simulink model "mod_liq2"  (R2016b)
settings: Solver=ode45  StartTime=0.0  StopTime=10.0  RelTol=1e-3  EnableMultiTasking=on
values from neighbouring files (symbols this model uses):
  Ar = 6*25.4    (= 152.4)    [param2NL.m]
  hmax = 16    [param2NL.m]
  k12 = 38    [param2NL.m]
  k2 = 11.5    [param2NL.m]
  qmax = 90    [param2NL.m]
  qmin = 0    [param2NL.m]
settings Model: Creator=Adolfo  LastModifiedBy=adolfobs
settings DataIOCC: LimitDataPoints=on  SaveFormat=Array  SignalLoggingSaveFormat=ModelDataLogs
settings OptimizationCC: ExpressionDepthLimit=2147483647  LifeSpan=inf
settings DebuggingCC: UnderspecifiedInitializationDetection=Classic  MergeDetectMultiDrivingBlocksExec=none  SolverPrmCheckMsg=warning  FcnCallInpInsideContextMsg=warning  StateNameClashWarn=warning  SFUnexpectedBacktrackingDiag=warning  SFNoUnconditionalDefaultTransitionDiag=warning  SFExecutionAtInitializationDiag=none
settings HardwareCC: ProdBitPerPointer=32  ProdBitPerSizeT=32  ProdBitPerPtrDiffT=32  ProdLargestAtomicFloat=None  ProdIntDivRoundTo=Undefined  ProdEndianess=Unspecified  ProdWordSize=32  ProdHWDeviceType=32-bit Generic
settings ModelReferenceCC: PropagateSignalLabelsOutOfModel=off
settings GRTTargetCC: TargetLangStandard=C89/C90 (ANSI)  GeneratePreprocessorConditionals=Disable all  CombineOutputUpdateFcns=off  GRTInterface=on
settings ConfigComp: CovMetricSettings=dw  CovHtmlReporting=on  CovSaveCumulativeToWorkspaceVar=on  CovSaveSingleToWorkspaceVar=on  CovExternalEMLEnable=off

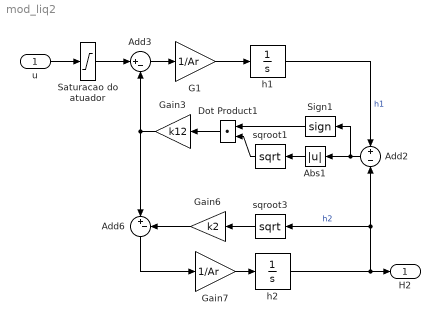
== system mod_liq2 ==
  u : Inport
  Abs1 : Abs
  Add2 : Sum  Inputs=+-
  Add3 : Sum  Inputs=|+-
  Add6 : Sum  Inputs=|+-
  Dot Product1 : DotProduct  InputSameDT=on  OutDataTypeStr=Inherit: Inherit via internal rule
  G1 : Gain  Gain=1/Ar
  Gain3 : Gain  Gain=k12
  Gain6 : Gain  Gain=k2
  Gain7 : Gain  Gain=1/Ar
  Saturacao do atuador : Saturate  UpperLimit=qmax  LowerLimit=qmin
  Sign1 : Signum
  h1 : Integrator  LimitOutput=on  UpperSaturationLimit=hmax  LowerSaturationLimit=0
  h2 : Integrator  LimitOutput=on  UpperSaturationLimit=hmax  LowerSaturationLimit=0
  sqroot1 : Math  Operator=sqrt  SaturateOnIntegerOverflow=on
  sqroot3 : Math  Operator=sqrt  SaturateOnIntegerOverflow=on
  H2 : Outport
  wires:
  h1/1 -> Add2/1  "h1"
  h2/1 -> H2/1, sqroot3/1, Add2/2  "h2"
  Saturacao do atuador/1 -> Add3/1
  Add6/1 -> Gain7/1
  Gain6/1 -> Add6/2
  Gain7/1 -> h2/1
  sqroot3/1 -> Gain6/1
  G1/1 -> h1/1
  Gain3/1 -> Add3/2, Add6/1
  Add3/1 -> G1/1
  Dot Product1/1 -> Gain3/1
  sqroot1/1 -> Dot Product1/2
  Sign1/1 -> Dot Product1/1
  Abs1/1 -> sqroot1/1
  Add2/1 -> Sign1/1, Abs1/1
  u/1 -> Saturacao do atuador/1
